simulink model "sl_puma"  (R2018b)
settings: Solver=ode45  StartTime=0.0  StopTime=time(end-1)  FixedStep=.001  RelTol=1e-3  EnableMultiTasking=on
values from neighbouring files (symbols this model uses):
  Kd = -eye(6)    [p560_startup_script.m]
  Kp = eye(6)    [p560_startup_script.m]
  traj = gen_traj()    [p560_startup_script.m]
undefined symbols (not defined in the file or in its folder): time
libraries: roblocks x2
settings Model: ExtModeTrigMode=oneshot  ExtModeArmWhenConnect=off  Creator=pic  LastModifiedBy=devon
settings DataIOCC: SaveFormat=Array  SignalLoggingSaveFormat=ModelDataLogs  SignalLogging=off  ReturnWorkspaceOutputs=on
settings OptimizationCC: BlockReduction=off  BooleanDataType=off  ExpressionDepthLimit=2147483647  InitFltsAndDblsToZero=on  LifeSpan=inf
settings DebuggingCC: SaveWithParameterizedLinksMsg=none  UnderspecifiedInitializationDetection=Classic  MergeDetectMultiDrivingBlocksExec=none  SignalResolutionControl=TryResolveAllWithWarning  MultiTaskDSMMsg=warning  MultiTaskCondExecSysMsg=none  FcnCallInpInsideContextMsg=warning  StateNameClashWarn=warning  SFUnexpectedBacktrackingDiag=warning  SFNoUnconditionalDefaultTransitionDiag=warning  SFExecutionAtInitializationDiag=none
settings HardwareCC: ProdBitPerPointer=32  ProdBitPerSizeT=32  ProdBitPerPtrDiffT=32  ProdLargestAtomicFloat=None  ProdIntDivRoundTo=Undefined  ProdEndianess=Unspecified  ProdWordSize=32  ProdHWDeviceType=32-bit Generic  TargetUnknown=on
settings ModelReferenceCC: PropagateSignalLabelsOutOfModel=off
settings SFSimCC: SimUseLocalCustomCode=off
settings RTWCC: RTWUseLocalCustomCode=off
settings CodeAppCC: StateflowObjectComments=on
settings GRTTargetCC: TargetLangStandard=C89/C90 (ANSI)  ModelReferenceCompliant=off  ParMdlRefBuildCompliant=off  CompOptLevelCompliant=off  GeneratePreprocessorConditionals=Disable all  CombineOutputUpdateFcns=off  MatFileLogging=off  GRTInterface=on
settings ConfigComp: CovMetricSettings=dw  CovHtmlReporting=on  CovSaveCumulativeToWorkspaceVar=on  CovSaveSingleToWorkspaceVar=on  CovExternalEMLEnable=off  CovSFcnEnable=off

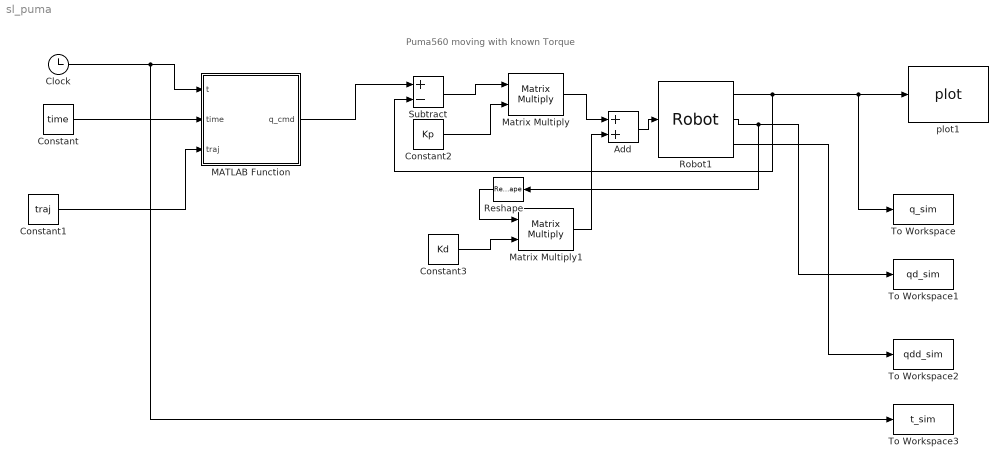
== system sl_puma ==
  note: Puma560 moving with known Torque
  Add : Sum
  Clock : Clock
  Constant : Constant  Value=time
  Constant1 : Constant  Value=traj
  Constant2 : Constant  Value=Kp
  Constant3 : Constant  Value=Kd
  MATLAB Function : MATLAB Function  TreatAsAtomicUnit=on
  Matrix Multiply : Product  Multiplication=Matrix(*)
  Matrix Multiply1 : Product  Multiplication=Matrix(*)
  Reshape : Reshape  OutputDimensionality=Row vector (2-D)
  Robot1 : roblocks/Arm/Robot  robot=p560  q0=[0 0 0 0 0 0]
  Subtract : Sum  Inputs=+-
  To Workspace : ToWorkspace  VariableName=q_sim  SampleTime=-1
  To Workspace1 : ToWorkspace  VariableName=qd_sim  SampleTime=-1
  To Workspace2 : ToWorkspace  VariableName=qdd_sim  SampleTime=-1
  To Workspace3 : ToWorkspace  VariableName=t_sim  SampleTime=-1
  plot1 : roblocks/Arm/plot  robot=p560  fps=5  holdplot=on
  wires:
  Robot1/1 -> Subtract/2, plot1/1, To Workspace/1
  Robot1/3 -> To Workspace2/1
  Robot1/2 -> Reshape/1, To Workspace1/1
  Clock/1 -> To Workspace3/1, MATLAB Function/1(t)
  Constant/1 -> MATLAB Function/2(time)
  Constant1/1 -> MATLAB Function/3(traj)
  MATLAB Function/1(q_cmd) -> Subtract/1
  Constant2/1 -> Matrix Multiply/2
  Subtract/1 -> Matrix Multiply/1
  Constant3/1 -> Matrix Multiply1/2
  Add/1 -> Robot1/1
  Matrix Multiply1/1 -> Add/2
  Matrix Multiply/1 -> Add/1
  Reshape/1 -> Matrix Multiply1/1

== matlab function sl_puma/MATLAB Function ==
  data: t input; q_cmd output; time input; traj input
function q_cmd = get_traj(t, time, traj)

q_cmd = interp1(time, traj, t);

end
